simulink model "SuspenseSystem"  (Simulink 10.0)
settings: Solver=VariableStepAuto  StartTime=0.0  StopTime=10.0  RelTol=1e-3
undefined symbols (not defined in the file): b, ks, kw, m1, m2
settings Model: Creator=aravind  LastModifiedBy=aravind
settings DataIOCC: SaveFormat=Dataset  ReturnWorkspaceOutputs=on
settings OptimizationCC: LifeSpan=auto
settings DebuggingCC: UnderspecifiedInitializationDetection=Simplified  MergeDetectMultiDrivingBlocksExec=error  SFUnexpectedBacktrackingDiag=error  SFNoUnconditionalDefaultTransitionDiag=error  SFExecutionAtInitializationDiag=warning  ArithmeticOperatorsInVariantConditions=error
settings HardwareCC: ProdBitPerPointer=64  ProdBitPerSizeT=64  ProdBitPerPtrDiffT=64  ProdLargestAtomicFloat=Float  ProdIntDivRoundTo=Zero  ProdEndianess=LittleEndian  ProdWordSize=64  ProdHWDeviceType=Intel->x86-64 (Windows64)
settings ModelReferenceCC: PropagateSignalLabelsOutOfModel=on
settings SFSimCC: SimUseLocalCustomCode=on  CustomCodeUndefinedFunction=FilterOut
settings RTWCC: RTWUseLocalCustomCode=on
settings CodeAppCC: StateflowObjectComments=off
settings GRTTargetCC: TargetLangStandard=C99 (ISO)  CombineOutputUpdateFcns=on  GRTInterface=off
settings ConfigComp: CovMetricSettings=dwe  CovHtmlReporting=off  CovSaveCumulativeToWorkspaceVar=off  CovSaveSingleToWorkspaceVar=off

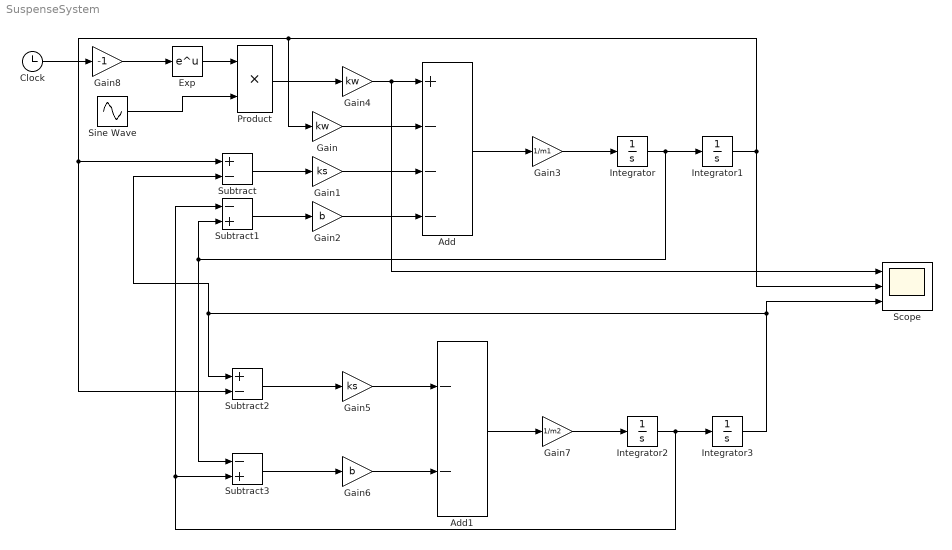
== system SuspenseSystem ==
  Add : Sum  Inputs=+---
  Add1 : Sum  Inputs=--
  Clock : Clock
  Exp : Math  SignedPower=off  SaturateOnIntegerOverflow=on
  Gain : Gain  Gain=kw
  Gain1 : Gain  Gain=ks
  Gain2 : Gain  Gain=b
  Gain3 : Gain  Gain=1/m1
  Gain4 : Gain  Gain=kw
  Gain5 : Gain  Gain=ks
  Gain6 : Gain  Gain=b
  Gain7 : Gain  Gain=1/m2
  Gain8 : Gain  Gain=-1
  Integrator{,1..3} (4 alike) : Integrator
  Product : Product
  Scope : Scope  NumInputPorts=3
  Sine Wave : Sin  Amplitude=10  SampleTime=0
  Subtract : Sum  Inputs=+-
  Subtract1 : Sum  Inputs=-+
  Subtract2 : Sum  Inputs=+-
  Subtract3 : Sum  Inputs=-+
  wires:
  Gain/1 -> Add/2
  Gain1/1 -> Add/3
  Gain2/1 -> Add/4
  Add/1 -> Gain3/1
  Gain3/1 -> Integrator/1
  Integrator1/1 -> Scope/2, Subtract2/2, Subtract/1, Gain/1
  Integrator/1 -> Subtract3/1, Subtract1/2, Integrator1/1
  Add1/1 -> Gain7/1
  Integrator2/1 -> Integrator3/1, Subtract1/1, Subtract3/2
  Gain7/1 -> Integrator2/1
  Integrator3/1 -> Scope/3, Subtract/2, Subtract2/1
  Gain6/1 -> Add1/2
  Gain5/1 -> Add1/1
  Subtract/1 -> Gain1/1
  Subtract1/1 -> Gain2/1
  Subtract2/1 -> Gain5/1
  Subtract3/1 -> Gain6/1
  Sine Wave/1 -> Product/2
  Exp/1 -> Product/1
  Gain4/1 -> Scope/1, Add/1
  Product/1 -> Gain4/1
  Gain8/1 -> Exp/1
  Clock/1 -> Gain8/1
